simulink model "MatlabfilePvsolar"  (R2024b)
settings: Solver=ode23tb  StartTime=0.0  StopTime=2  RelTol=1e-3
libraries: spsSeriesRLCBranchLib x4, spsCurrentMeasurementLib x2, spsDiodeLib x2, spsVoltageMeasurementLib x2, spsMosfetLib x1, spspowerguiLib x1, spsPVArrayLib x1, spsPWMGeneratorDCDCLib x1
settings Model: Creator=Meenu  LastModifiedBy=priya vaid

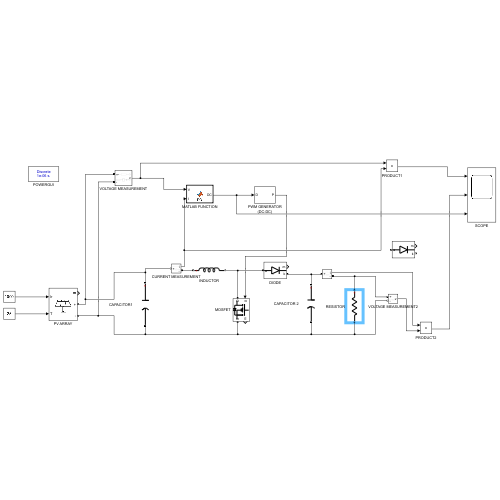
[thumbnail: Simulink's stored preview of the top-level diagram]
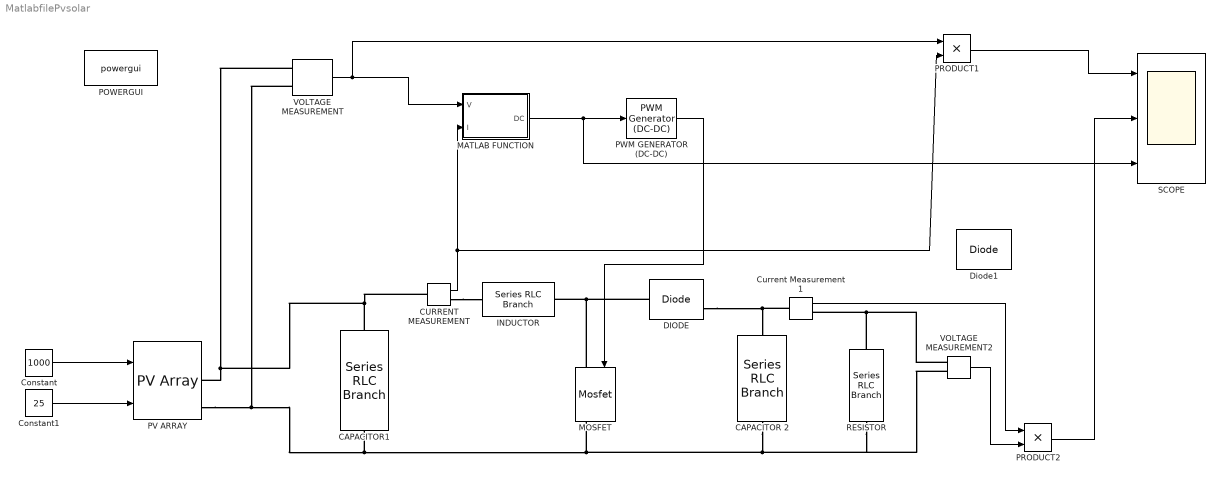
== system MatlabfilePvsolar ==
  CAPACITOR 2 : spsSeriesRLCBranchLib/Series RLC Branch  LConnTagsString=__new0  RConnTagsString=__new0  BranchType=C  Resistance=1  Inductance=1e-3  SetiL0=off  InitialCurrent=0  Capacitance=100e-6  Setx0=off  InitialVoltage=0  Measurements=None
  CAPACITOR1 : spsSeriesRLCBranchLib/Series RLC Branch  LConnTagsString=__new0  RConnTagsString=__new0  BranchType=C  Resistance=1  Inductance=1e-3  SetiL0=off  InitialCurrent=0  Capacitance=20e-6  Setx0=off  InitialVoltage=0  Measurements=None
  CURRENT MEASUREMENT : spsCurrentMeasurementLib/Current Measurement  PhasorSimulation=off  OutputType=Complex  PSBequivalent=0
  Constant : Constant  Value=1000
  Constant1 : Constant  Value=25
  Current Measurement1 : spsCurrentMeasurementLib/Current Measurement  PhasorSimulation=off  OutputType=Complex  PSBequivalent=0
  DIODE : spsDiodeLib/Diode  Ron=0.001  Lon=0  Vf=0  IC=0  UseSnubber=0  Rs=inf  Cs=inf  Measurements=on
  Diode1 : spsDiodeLib/Diode  Ron=0.001  Lon=0  Vf=0.8  IC=0  UseSnubber=0  Rs=inf  Cs=inf  Measurements=on
  INDUCTOR : spsSeriesRLCBranchLib/Series RLC Branch  LConnTagsString=__new0  RConnTagsString=__new0  BranchType=L  Resistance=1  Inductance=10e-3  SetiL0=off  InitialCurrent=0  Capacitance=1e-6  Setx0=off  InitialVoltage=0  Measurements=None
  MATLAB FUNCTION : MATLAB Function  TreatAsAtomicUnit=on
  MOSFET : spsMosfetLib/Mosfet  Ron=0.1  Lon=0  Rd=0.01  Vfd=0  IC=0  Rs=1e5  Cs=inf  Measurements=on
  POWERGUI : spspowerguiLib/powergui  Priority=1  SimulationMode=Discrete  SampleTime=1e-6  frequency=60  Iterations=50  frequencyindice=0  Pbase=100e6  ErrMax=1e-4  UnitsV=kV  UnitsW=MW  buscounter=0  FunctionMessages=off  echomessages=off  EnableUseOfTLC=off  CurrentSourceSwitches=off  DisableSnubberDevices=off  DisableRonSwitches=off  DisableVfSwitches=off  DisplayEquations=off  AutomaticDiscreteSolvers=off  SolverType=Tustin/Backward Euler (TBE)  Interpol=off  ExternalGateDelay=off  methode=off  Ts=100  x0status=blocks  SPID=on  SwTol=0  HookPort=off  NonlinearTolerance=1e-4  nMaxIteration=100  ContinueOnMaxIteration=off  RestoreLinks=warning  ResistiveCurrentMeasurement=off  Frange=[0:2:500]  Ylog=off  Xlog=on  ShowGrid=off  save=off  variable=ZData  structure=0  ZoomFFT=off  StartTime=0.0  cycles=1  DisplayStyle=1  fundamental=60  FreqAxis=off  MaxFrequency=1000  frequencyindicesteady=1  RmsSteady=1  display=off
  PRODUCT1 : Product
  PRODUCT2 : Product
  PV ARRAY : spsPVArrayLib/PV Array  Npar=1  Nser=1  PlotType=array @ 25 deg.C & specified irradiances  S_vec="[ 1000  600  100 ]"  Temp_C_vec="[ 45 25  ]"  ModuleName=User-defined  PlotWhenSelected=off  Pm=120  Ncell=60  Voc=75  Isc=2.4  Vm=60  Im=2  beta_Voc_pc=-0.36099  alpha_Isc_pc=0.102  beta_Voc=-0.27074  alpha_Isc=0.002448  IL=2.4337  I0=8.6067e-11  nI=2.0362  Rsh=195.7758  Rs=2.7456  RobustModel=off  RobustCellTemperature=313.3991  BAL=on  Tc=1e-6  Tfilter=5e-5
  PWM GENERATOR (DC-DC) : spsPWMGeneratorDCDCLib/PWM Generator (DC-DC)  Fsw=25000  Ts=0
  RESISTOR : spsSeriesRLCBranchLib/Series RLC Branch  LConnTagsString=__new0  RConnTagsString=__new0  BranchType=R  Resistance=120  Inductance=1e-3  SetiL0=off  InitialCurrent=0  Capacitance=100e-6  Setx0=off  InitialVoltage=0  Measurements=None
  SCOPE : Scope  NumInputPorts=3
  VOLTAGE MEASUREMENT : spsVoltageMeasurementLib/Voltage Measurement  PhasorSimulation=off  OutputType=Complex  PSBequivalent=0
  VOLTAGE MEASUREMENT2 : spsVoltageMeasurementLib/Voltage Measurement  PhasorSimulation=off  OutputType=Complex  PSBequivalent=0
  wires:
  Constant/1 -> PV ARRAY/1
  Constant1/1 -> PV ARRAY/2
  VOLTAGE MEASUREMENT/1 -> PRODUCT1/1, MATLAB FUNCTION/1(V)
  CURRENT MEASUREMENT/1 -> MATLAB FUNCTION/2(I), PRODUCT1/2
  MATLAB FUNCTION/1(DC) -> SCOPE/3, PWM GENERATOR (DC-DC)/1
  PWM GENERATOR (DC-DC)/1 -> MOSFET/1
  Current Measurement1/1 -> PRODUCT2/1
  VOLTAGE MEASUREMENT2/1 -> PRODUCT2/2
  PRODUCT2/1 -> SCOPE/2
  PRODUCT1/1 -> SCOPE/1
  connections:
  CAPACITOR1/LConn1 -- CURRENT MEASUREMENT/LConn1 -- PV ARRAY/RConn1 -- VOLTAGE MEASUREMENT/LConn1
  PV ARRAY/RConn2 -- VOLTAGE MEASUREMENT/LConn2 -- VOLTAGE MEASUREMENT2/LConn2 -- RESISTOR/RConn1 -- CAPACITOR 2/RConn1 -- MOSFET/RConn1 -- CAPACITOR1/RConn1
  DIODE/LConn1 -- MOSFET/LConn1 -- INDUCTOR/RConn1
  DIODE/RConn1 -- Current Measurement1/LConn1 -- CAPACITOR 2/LConn1
  CURRENT MEASUREMENT/RConn1 -- INDUCTOR/LConn1
  RESISTOR/LConn1 -- VOLTAGE MEASUREMENT2/LConn1 -- Current Measurement1/RConn1

== matlab function MatlabfilePvsolar/MATLAB FUNCTION ==
  data: V input; DC output; I input
function DC = PO(V,I) %fitness function
persistent countP1 Ppr Pcu Vpr Vcu Dcu Dpr deltaD;
if(isempty(countP1))
 countP1=0;
 Ppr=0;
 Pcu=0;
 Vpr=0;
 Vcu=0;
 Dcu=0;
 Dpr=0.16;
 deltaD=0.02;
end
countP1=countP1+1;
if(countP1>=1 && countP1<5000)
 Dcu=Dpr
elseif(countP1==5000)
 Pcu=V*I;
 Vcu=V;
 if(Pcu-Ppr>0)
 if(Vcu-Vpr>0)
 Dcu=Dpr-deltaD;
 elseif(Vcu-Vpr<0)
 Dcu=Dpr+deltaD;
 end
 elseif(Pcu-Ppr<0)
 if(Vcu-Vpr>0)
 Dcu=Dpr+deltaD

 elseif(Vcu-Vpr<0)
 Dcu=Dpr-deltaD
 end

 elseif(Pcu-Ppr==0)
 Dcu=Dpr
 end
elseif (countP1==5001)
Dpr=Dcu
Vpr=Vcu
Ppr=Pcu
countP1=0;
end
DC=Dcu
